simulink model "lineardesign"  (R2016a)
settings: Solver=ode45  StartTime=0.0  StopTime=10  RelTol=1e-3
values from neighbouring files (symbols this model uses):
  K = lqr(A,B,Q,R)    [lindesign.m]
  z0 = [q10;q20;q1dot0;q2dot0]    [lindesign.m]
  zeq = [0;pi/2;0;0]    [lindesign.m]
undefined symbols (not defined in the file or in its folder): cartpend
settings Model: Creator=rhanz  LastModifiedBy=rhanz
settings DataIOCC: LimitDataPoints=on  SaveFormat=Array  SignalLoggingSaveFormat=ModelDataLogs
settings OptimizationCC: ExpressionDepthLimit=2147483647
settings DebuggingCC: UnderspecifiedInitializationDetection=Classic  MergeDetectMultiDrivingBlocksExec=none  SolverPrmCheckMsg=warning  FcnCallInpInsideContextMsg=UseLocalSettings  StateNameClashWarn=warning
settings HardwareCC: ProdBitPerPointer=32  ProdLargestAtomicFloat=None  ProdIntDivRoundTo=Undefined  ProdEndianess=Unspecified  ProdWordSize=32  ProdHWDeviceType=32-bit Generic
settings ModelReferenceCC: PropagateSignalLabelsOutOfModel=off
settings GRTTargetCC: CombineOutputUpdateFcns=off  GRTInterface=on
settings ConfigComp: CovModelRefEnable=Off

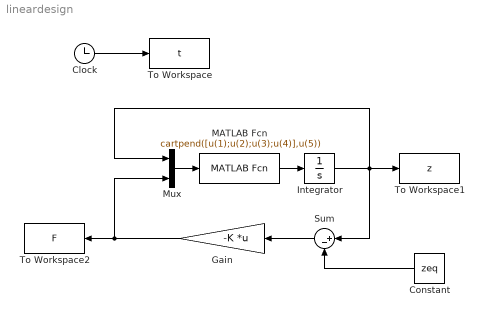
== system lineardesign ==
  Clock : Clock
  Constant : Constant  Value=zeq
  Gain : Gain  Gain=-K  Multiplication=Matrix(K*u) (u vector)
  Integrator : Integrator  InitialCondition=z0
  MATLAB Fcn : MATLABFcn  MATLABFcn=cartpend([u(1);u(2);u(3);u(4)],u(5))
  Mux : Mux  Inputs=2
  Sum : Sum  Inputs=|+-
  To Workspace : ToWorkspace  VariableName=t  SampleTime=-1
  To Workspace1 : ToWorkspace  VariableName=z  SampleTime=-1
  To Workspace2 : ToWorkspace  VariableName=F  SampleTime=-1
  wires:
  MATLAB Fcn/1 -> Integrator/1
  Mux/1 -> MATLAB Fcn/1
  Gain/1 -> Mux/2, To Workspace2/1
  Integrator/1 -> Sum/1, Mux/1, To Workspace1/1
  Clock/1 -> To Workspace/1
  Constant/1 -> Sum/2
  Sum/1 -> Gain/1
